simulink model "model_temperature"  (R2022b)
settings: Solver=VariableStepAuto  StartTime=0.0  StopTime=20  RelTol=1e-3
settings Model: Creator=mateo  LastModifiedBy=mateo

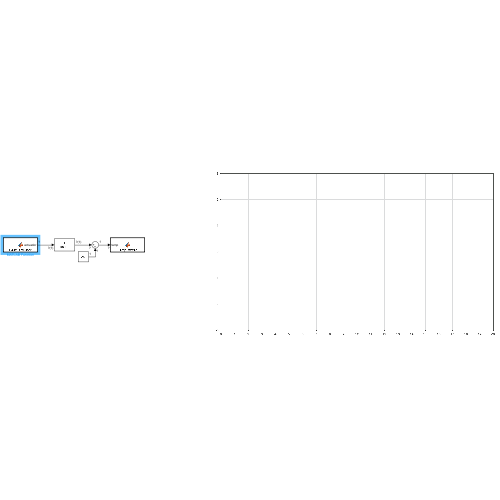
[thumbnail: Simulink's stored preview of the top-level diagram]
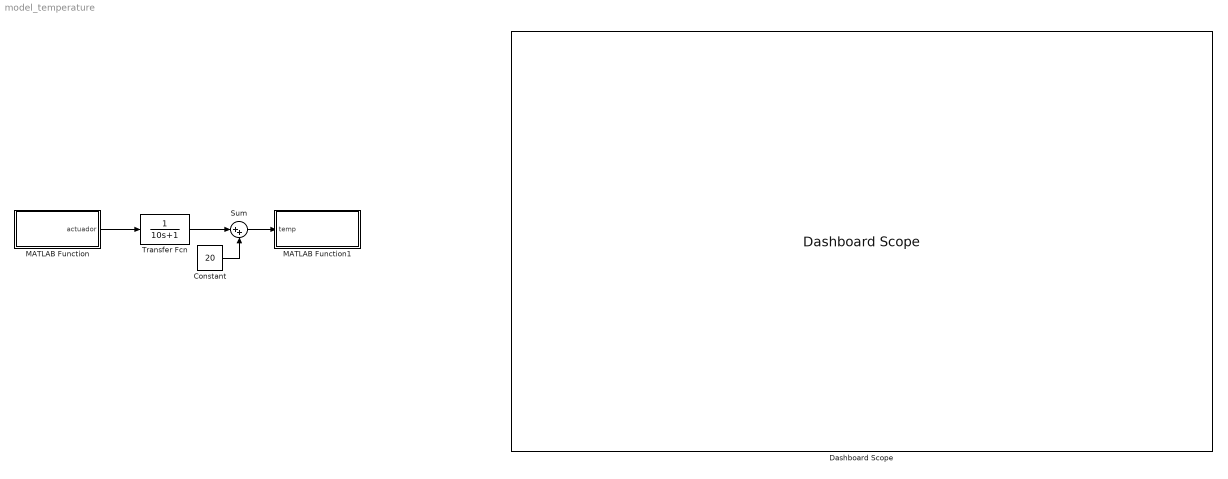
== system model_temperature ==
  Constant : Constant  Value=20
  Dashboard Scope : DashboardScope
  MATLAB Function : MATLAB Function  TreatAsAtomicUnit=on
  MATLAB Function1 : MATLAB Function  TreatAsAtomicUnit=on
  Sum : Sum  Inputs=|++
  Transfer Fcn : TransferFcn  Denominator=[10 1]
  wires:
  MATLAB Function/1(actuador) -> Transfer Fcn/1
  Transfer Fcn/1 -> Sum/1
  Constant/1 -> Sum/2
  Sum/1 -> MATLAB Function1/1(temp)

== matlab function model_temperature/MATLAB Function ==
  data: actuador output
function actuador = Heat_actuator()
    client = modbus("tcpip","192,168.10.7",502);
    actuador=read(client,"inputregs",1,1)

== matlab function model_temperature/MATLAB Function1 ==
  data: temp input
function Temp_writer(temp)
    client = modbus("tcpip","192,168.10.7",502);
    write(client,"holdingregs",2,round(temp));
